simulink model "regulacjapogodowaobiekt"  (R2022b)
settings: Solver=VariableStepAuto  StartTime=0.0  StopTime=tmax  MaxStep=2  RelTol=1e-3
undefined symbols (not defined in the file): ap_gz, ap_wz, az_gz, az_wz, bp_gz, bp_wz, bz_gz, bz_wz, Cpw, Cvg, Cvo1, Cvo2, Cvw, dFmg1, dFmg2, dQt1, dQt2, dTwew1, dTzew, Fmg0, Fmw0, Kcg, Kco, Kcw, Ki, Kp, QtN, SumT0, T0, Tgp10, Tgp20, Tgz10, Tgz20, Ti, Toz0, tsok, Twew10, Twew20, TwewN, Twp0, Twz0, Tzew0
settings Model: Creator=asialalala  LastModifiedBy=asialalala
settings DataIOCC: ReturnWorkspaceOutputs=off

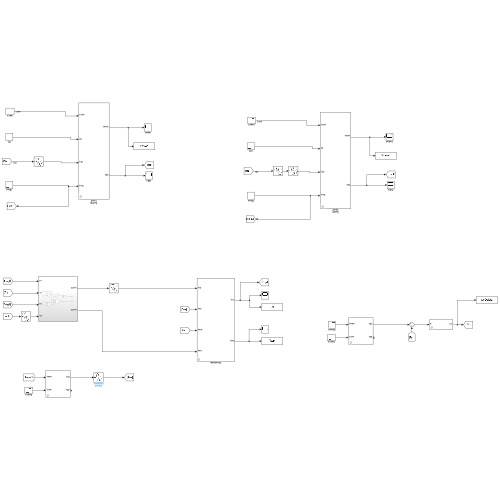
[thumbnail: Simulink's stored preview of the top-level diagram]
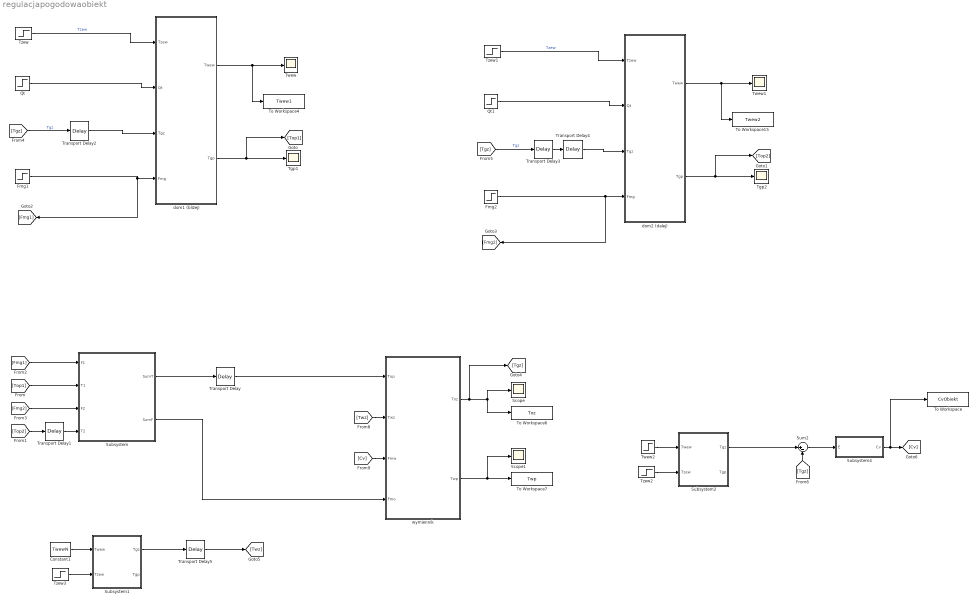
== system regulacjapogodowaobiekt ==
  Constant1 : Constant  Value=TwewN
  Fmg1 : Step  Time=tsok  Before=Fmg0  After=Fmg0 + dFmg1  SampleTime=0
  Fmg2 : Step  Time=tsok  Before=Fmg0  After=Fmg0 + dFmg2  SampleTime=0
  Qt : Step  Time=tsok  Before=QtN  After=QtN + dQt1  SampleTime=0
  Qt1 : Step  Time=tsok  Before=QtN  After=QtN + dQt2  SampleTime=0
  Scope : Scope
  Scope1 : Scope
  Subsystem : Subsystem
  Subsystem1 : Subsystem  mask{az=az_wz, bz=bz_wz, ap=ap_wz, bp=bp_wz}
  Subsystem2 : Subsystem  mask{az=az_gz, bz=bz_gz, ap=ap_gz, Parameter4=bp_gz}
      mask prompts: Parameter4 "bp"
  Subsystem4 : Subsystem  mask{Kp=Kp, Ti=Ti, Cv0=Fmw0, Ki=Ki}
  Sum2 : Sum  Inputs=|+-
  Tgp1 : Scope
  Tgp2 : Scope
  To Workspace : ToWorkspace  VariableName=CvObiekt  SampleTime=-1
  To Workspace15 : ToWorkspace  VariableName=Twew2  SampleTime=-1
  To Workspace4 : ToWorkspace  VariableName=Twew1  SampleTime=-1
  To Workspace6 : ToWorkspace  VariableName=Toz  SampleTime=-1
  To Workspace7 : ToWorkspace  VariableName=Twp  SampleTime=-1
  Transport Delay : TransportDelay  DelayTime=T0  InitialOutput=SumT0
  Transport Delay1 : TransportDelay  DelayTime=T0  InitialOutput=Tgp20
  Transport Delay2 : TransportDelay  DelayTime=T0  InitialOutput=Tgz10
  Transport Delay3 : TransportDelay  DelayTime=T0  InitialOutput=Tgz20
  Transport Delay4 : TransportDelay  DelayTime=T0  InitialOutput=Tgz20
  Transport Delay5 : TransportDelay  DelayTime=1200  InitialOutput=Twz0
  Twew : Scope
  Twew1 : Scope
  Twew2 : Step  Time=tsok  Before=Twew10  After=Twew10 + dTwew1  SampleTime=0
  Tzew{,1..3} (4 alike) : Step  Time=tsok  Before=Tzew0  After=Tzew0 + dTzew  SampleTime=0
  dom1 (bliżej) : Subsystem  mask{Kcw=Kcw, Kcg=Kcg, Cvw=Cvw, Cvg=Cvg, Cpw=Cpw}
  dom2 (dalej) : Subsystem  mask{Kcw=Kcw, Kcg=Kcg, Cvw=Cvw, Cvg=Cvg, Cpw=Cpw}
  wymiennik : Subsystem  mask{Cvo1=Cvo1, Cvo2=Cvo2, Kco=Kco}
  wires:
  Tzew/1 -> dom1 (bliżej)/1(Tzew)  "Tzew"
  Qt/1 -> dom1 (bliżej)/2(Qt)
  dom1 (bliżej)/1(Twew) -> Twew/1, To Workspace4/1
  dom1 (bliżej)/2(Tgp) -> [Top1], Tgp1/1
  wymiennik/1(Toz) -> [Tgz], Scope/1, To Workspace6/1
  wymiennik/2(Twp) -> Scope1/1, To Workspace7/1
  Subsystem/1(SumT) -> Transport Delay/1
  Tzew1/1 -> dom2 (dalej)/1(Tzew)  "Tzew"
  dom2 (dalej)/2(Tgp) -> [Top2], Tgp2/1
  Qt1/1 -> dom2 (dalej)/2(Qt)
  dom2 (dalej)/1(Twew) -> Twew1/1, To Workspace15/1
  [Top1] -> Subsystem/2(T1)
  [Fmg1] -> Subsystem/1(F1)
  Subsystem/2(SumF) -> wymiennik/4(Fmo)
  [Fmg2] -> Subsystem/3(F2)
  Fmg1/1 -> [Fmg1], dom1 (bliżej)/4(Fmg)
  Fmg2/1 -> [Fmg2], dom2 (dalej)/4(Fmg)
  [Top2] -> Transport Delay1/1
  Transport Delay3/1 -> Transport Delay4/1
  [Tgz] -> Transport Delay2/1  "Tgz"
  Transport Delay2/1 -> dom1 (bliżej)/3(Tgz)
  Transport Delay4/1 -> dom2 (dalej)/3(Tgz)
  [Tgz] -> Transport Delay3/1  "Tgz"
  Transport Delay/1 -> wymiennik/1(Top)
  Transport Delay1/1 -> Subsystem/4(T2)
  Twew2/1 -> Subsystem2/1(Twew)
  Tzew2/1 -> Subsystem2/2(Tzew)
  Sum2/1 -> Subsystem4/1(E)
  Subsystem2/1(Tgz) -> Sum2/1
  [Tgz] -> Sum2/2
  Subsystem4/1(Cv) -> To Workspace/1, [Cv]
  Constant1/1 -> Subsystem1/1(Twew)
  Tzew3/1 -> Subsystem1/2(Tzew)
  Subsystem1/1(Tgz) -> Transport Delay5/1
  Transport Delay5/1 -> [Twz]
  [Twz] -> wymiennik/2(Twz)
  [Cv] -> wymiennik/3(Fmw)

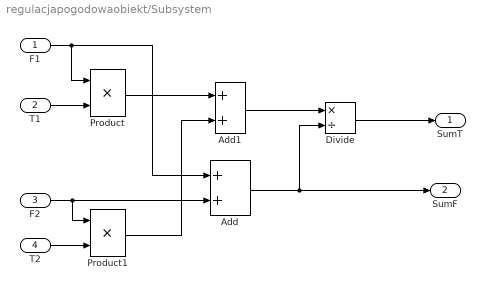
== system regulacjapogodowaobiekt/Subsystem ==
  F1 : Inport
  T1 : Inport  Port=2
  F2 : Inport  Port=3
  T2 : Inport  Port=4
  Add : Sum
  Add1 : Sum
  Divide : Product  Inputs=*/
  Product : Product
  Product1 : Product
  SumT : Outport
  SumF : Outport  Port=2
  wires:
  Add/1 -> Divide/2, SumF/1
  F2/1 -> Add/2, Product1/1
  F1/1 -> Product/1, Add/1
  T1/1 -> Product/2
  T2/1 -> Product1/2
  Product1/1 -> Add1/2
  Product/1 -> Add1/1
  Add1/1 -> Divide/1
  Divide/1 -> SumT/1

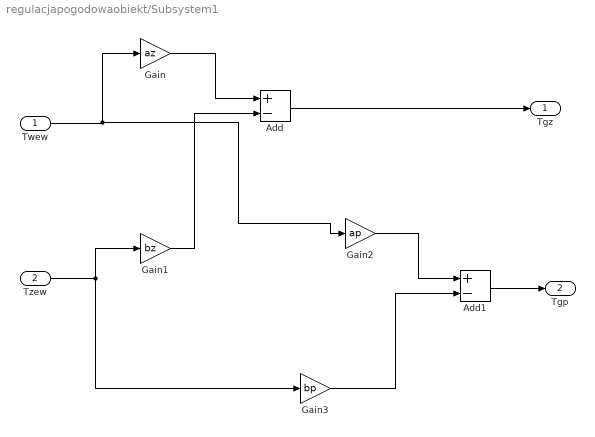
== system regulacjapogodowaobiekt/Subsystem1 ==
  Twew : Inport
  Tzew : Inport  Port=2
  Add : Sum  Inputs=+-
  Add1 : Sum  Inputs=+-
  Gain : Gain  Gain=az
  Gain1 : Gain  Gain=bz
  Gain2 : Gain  Gain=ap
  Gain3 : Gain  Gain=bp
  Tgz : Outport
  Tgp : Outport  Port=2
  wires:
  Gain1/1 -> Add/2
  Gain/1 -> Add/1
  Add/1 -> Tgz/1
  Add1/1 -> Tgp/1
  Twew/1 -> Gain2/1, Gain/1
  Gain2/1 -> Add1/1
  Tzew/1 -> Gain3/1, Gain1/1
  Gain3/1 -> Add1/2

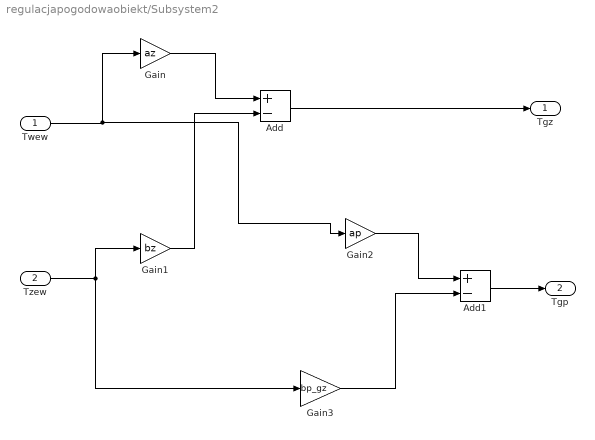
== system regulacjapogodowaobiekt/Subsystem2 ==
  Twew : Inport
  Tzew : Inport  Port=2
  Add : Sum  Inputs=+-
  Add1 : Sum  Inputs=+-
  Gain : Gain  Gain=az
  Gain1 : Gain  Gain=bz
  Gain2 : Gain  Gain=ap
  Gain3 : Gain  Gain=bp_gz
  Tgz : Outport
  Tgp : Outport  Port=2
  wires:
  Gain1/1 -> Add/2
  Gain/1 -> Add/1
  Add/1 -> Tgz/1
  Add1/1 -> Tgp/1
  Twew/1 -> Gain2/1, Gain/1
  Gain2/1 -> Add1/1
  Tzew/1 -> Gain3/1, Gain1/1
  Gain3/1 -> Add1/2

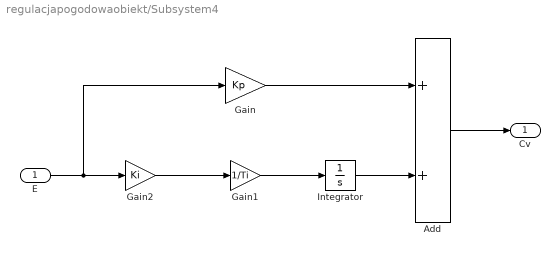
== system regulacjapogodowaobiekt/Subsystem4 ==
  E : Inport
  Add : Sum
  Gain : Gain  Gain=Kp
  Gain1 : Gain  Gain=1/Ti
  Gain2 : Gain  Gain=Ki
  Integrator : Integrator  InitialCondition=Cv0
  Cv : Outport
  wires:
  E/1 -> Gain/1, Gain2/1
  Gain2/1 -> Gain1/1
  Gain1/1 -> Integrator/1
  Add/1 -> Cv/1
  Gain/1 -> Add/1
  Integrator/1 -> Add/2

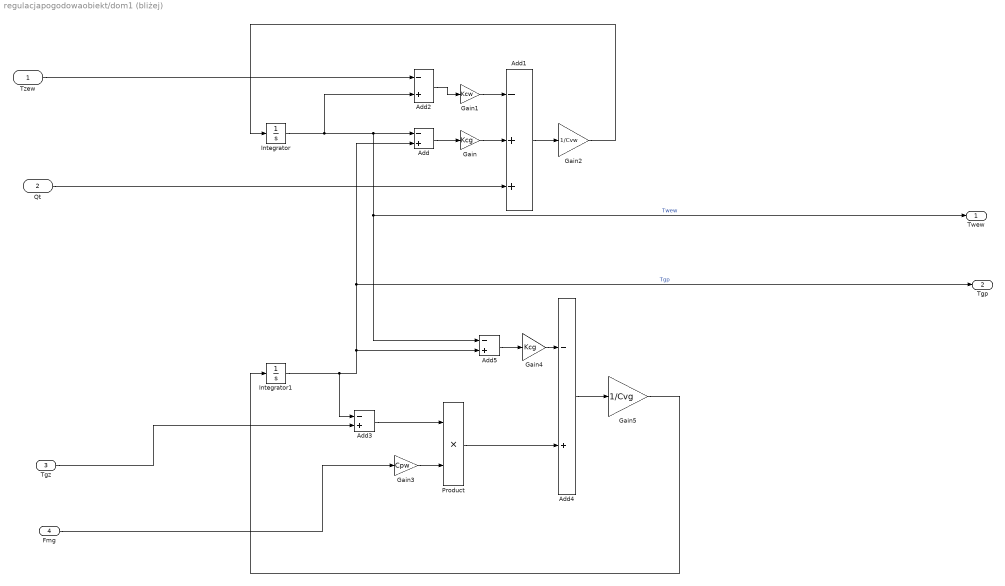
== system regulacjapogodowaobiekt/dom1 (bliżej) ==
  Tzew : Inport
  Qt : Inport  Port=2
  Tgz : Inport  Port=3
  Fmg : Inport  Port=4
  Add{,2..5} (5 alike) : Sum  Inputs=-+
  Add1 : Sum  Inputs=-++
  Gain : Gain  Gain=Kcg
  Gain1 : Gain  Gain=Kcw
  Gain2 : Gain  Gain=1/Cvw
  Gain3 : Gain  Gain=Cpw
  Gain4 : Gain  Gain=Kcg
  Gain5 : Gain  Gain=1/Cvg
  Integrator : Integrator  InitialCondition=Twew10
  Integrator1 : Integrator  InitialCondition=Tgp10
  Product : Product
  Twew : Outport
  Tgp : Outport  Port=2
  wires:
  Fmg/1 -> Gain3/1
  Add/1 -> Gain/1
  Gain3/1 -> Product/2
  Qt/1 -> Add1/3
  Product/1 -> Add4/2
  Gain2/1 -> Integrator/1
  Add2/1 -> Gain1/1
  Add5/1 -> Gain4/1
  Integrator1/1 -> Add3/1, Add5/2, Tgp/1, Add/2  "Tgp"
  Integrator/1 -> Add2/2, Twew/1, Add5/1, Add/1  "Twew"
  Gain/1 -> Add1/2
  Gain4/1 -> Add4/1
  Gain1/1 -> Add1/1
  Tzew/1 -> Add2/1
  Add3/1 -> Product/1
  Gain5/1 -> Integrator1/1
  Add4/1 -> Gain5/1
  Add1/1 -> Gain2/1
  Tgz/1 -> Add3/2

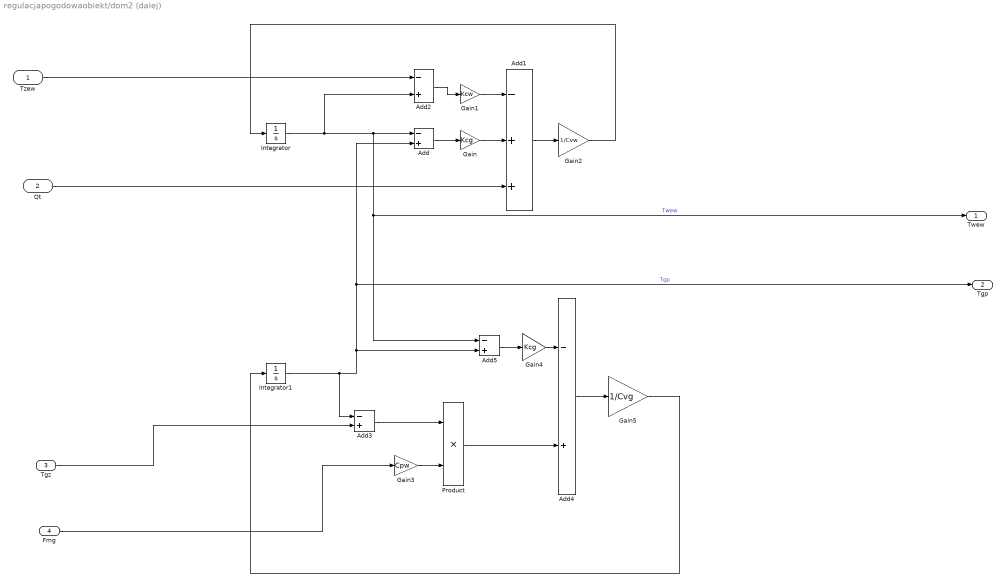
== system regulacjapogodowaobiekt/dom2 (dalej) ==
  Tzew : Inport
  Qt : Inport  Port=2
  Tgz : Inport  Port=3
  Fmg : Inport  Port=4
  Add{,2..5} (5 alike) : Sum  Inputs=-+
  Add1 : Sum  Inputs=-++
  Gain : Gain  Gain=Kcg
  Gain1 : Gain  Gain=Kcw
  Gain2 : Gain  Gain=1/Cvw
  Gain3 : Gain  Gain=Cpw
  Gain4 : Gain  Gain=Kcg
  Gain5 : Gain  Gain=1/Cvg
  Integrator : Integrator  InitialCondition=Twew20
  Integrator1 : Integrator  InitialCondition=Tgp20
  Product : Product
  Twew : Outport
  Tgp : Outport  Port=2
  wires:
  Fmg/1 -> Gain3/1
  Add/1 -> Gain/1
  Gain3/1 -> Product/2
  Qt/1 -> Add1/3
  Product/1 -> Add4/2
  Gain2/1 -> Integrator/1
  Add2/1 -> Gain1/1
  Add5/1 -> Gain4/1
  Integrator1/1 -> Add3/1, Add5/2, Tgp/1, Add/2  "Tgp"
  Integrator/1 -> Add2/2, Twew/1, Add5/1, Add/1  "Twew"
  Gain/1 -> Add1/2
  Gain4/1 -> Add4/1
  Gain1/1 -> Add1/1
  Tzew/1 -> Add2/1
  Add3/1 -> Product/1
  Gain5/1 -> Integrator1/1
  Add4/1 -> Gain5/1
  Add1/1 -> Gain2/1
  Tgz/1 -> Add3/2

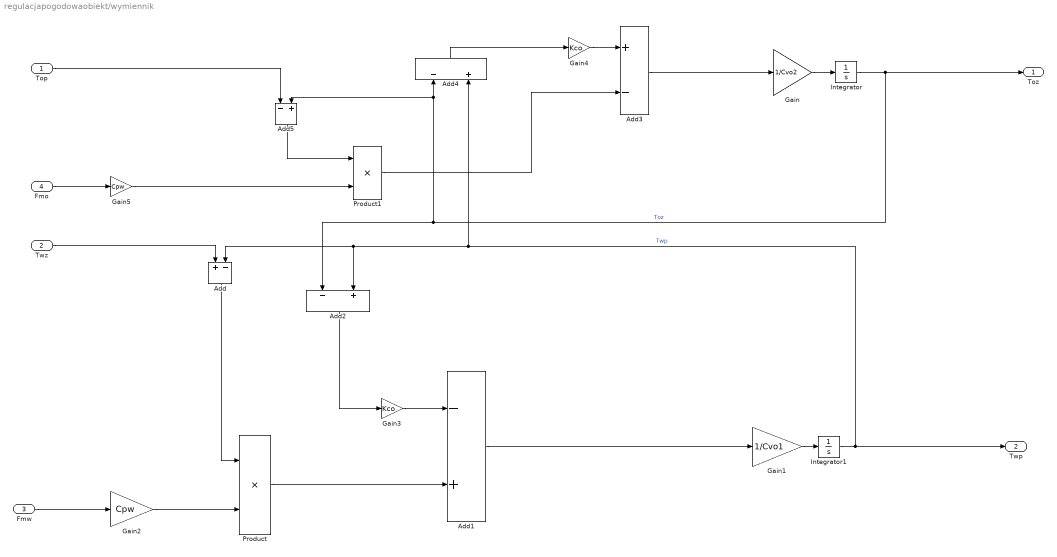
== system regulacjapogodowaobiekt/wymiennik ==
  Top : Inport
  Twz : Inport  Port=2
  Fmw : Inport  Port=3
  Fmo : Inport  Port=4
  Add : Sum  Inputs=+-
  Add{1..2,4..5} (4 alike) : Sum  Inputs=-+
  Add3 : Sum  Inputs=+-
  Gain : Gain  Gain=1/Cvo2
  Gain1 : Gain  Gain=1/Cvo1
  Gain2 : Gain  Gain=Cpw
  Gain3 : Gain  Gain=Kco
  Gain4 : Gain  Gain=Kco
  Gain5 : Gain  Gain=Cpw
  Integrator : Integrator  InitialCondition=Toz0
  Integrator1 : Integrator  InitialCondition=Twp0
  Product : Product
  Product1 : Product
  Toz : Outport
  Twp : Outport  Port=2
  wires:
  Integrator/1 -> Add2/1, Add5/2, Add4/1, Toz/1  "Toz"
  Integrator1/1 -> Twp/1, Add/2, Add2/2, Add4/2  "Twp"
  Gain/1 -> Integrator/1
  Gain1/1 -> Integrator1/1
  Fmw/1 -> Gain2/1
  Twz/1 -> Add/1
  Gain2/1 -> Product/2
  Add/1 -> Product/1
  Product/1 -> Add1/2
  Gain3/1 -> Add1/1
  Add2/1 -> Gain3/1
  Add1/1 -> Gain1/1
  Add3/1 -> Gain/1
  Gain4/1 -> Add3/1
  Add4/1 -> Gain4/1
  Fmo/1 -> Gain5/1
  Gain5/1 -> Product1/2
  Add5/1 -> Product1/1
  Product1/1 -> Add3/2
  Top/1 -> Add5/1
